simulink model "lab2_model"  (R2025a)
settings: Solver=ode45  StartTime=0.0  StopTime=3  MaxStep=0.001  RelTol=1e-3
values from neighbouring files (symbols this model uses):
  A = [-6 -25; 1 0]    [lab2.m]
  B = [ 25; 0]    [lab2.m]
  C = [1 0; 0 1]    [lab2.m]
  D = [0;0]    [lab2.m]
settings Model: Creator=marksorial  LastModifiedBy=marksorial

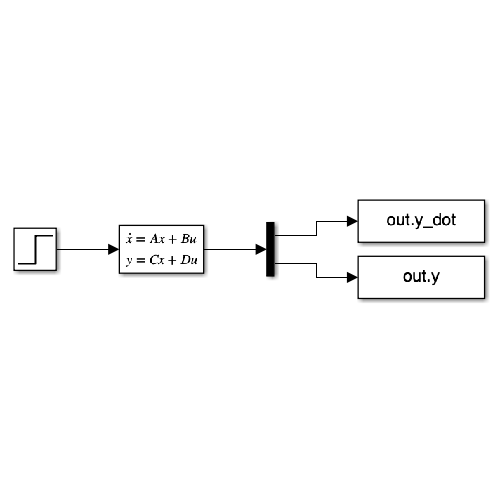
[thumbnail: Simulink's stored preview of the top-level diagram]
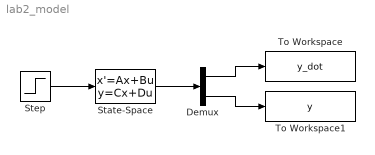
== system lab2_model ==
  Demux : Demux  Outputs=2
  State-Space : StateSpace  A=A  B=B  C=C  D=D  InitialCondition=0
  Step : Step  Time=0  SampleTime=0
  To Workspace : ToWorkspace  VariableName=y_dot  SampleTime=-1
  To Workspace1 : ToWorkspace  VariableName=y  SampleTime=-1
  wires:
  Step/1 -> State-Space/1
  State-Space/1 -> Demux/1
  Demux/1 -> To Workspace/1
  Demux/2 -> To Workspace1/1
